simulink model "SmartphoneBatteryRectifierModel"  (R2024a)
settings: Solver=ode23t  StartTime=0.0  StopTime=10  RelTol=1e-3
libraries: nesl_utility x8, fl_lib x6, ee_lib x4, batteryecm_lib x1
settings Model: Creator=callie  LastModifiedBy=callie
settings SimscapeCC: SimscapeLogType=all  SimscapeLogLimitData=off

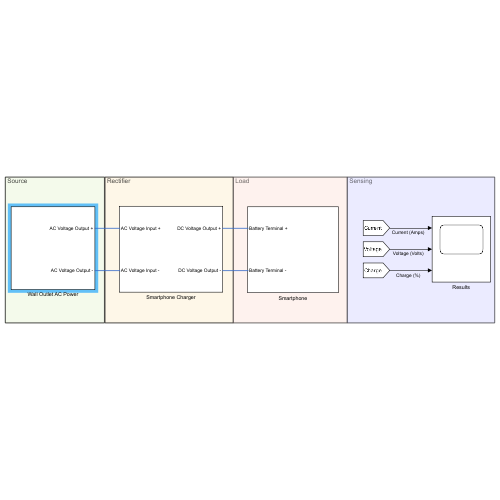
[thumbnail: Simulink's stored preview of the top-level diagram]
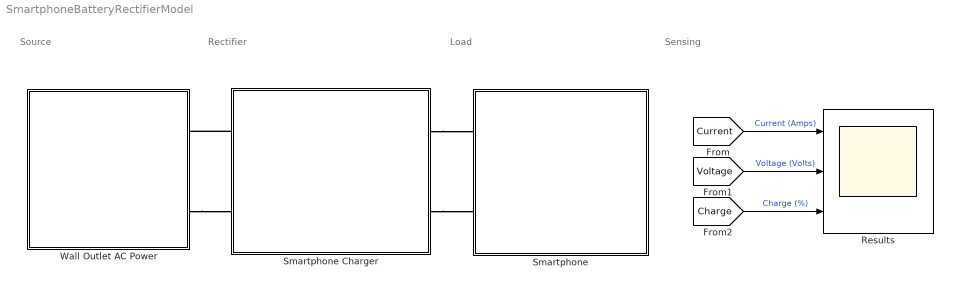
== system SmartphoneBatteryRectifierModel ==
  note: Sensing
  note: Load
  note: Rectifier
  note: Source
  Results : Scope  NumInputPorts=3
  Smartphone : Subsystem
      settings: PortSchema="{\"entries\":[{\"content\":{\"sides\":[{\"content\":{},\"type\":\"ConnectorPlacement.EquallySpacedRectSide\",\"uuid\":\"c6623932-9384-4505-9c8a-7aa7c6d03efe\"},{\"content\":{\"side\":\"RIGHT\"},\"type\":\"ConnectorPlacement.EquallySpacedRectSide\",\"uuid\":\"b63081fa-6f2e-4d52-89b7-0b15c2ff5a8a\"},{\"content\":{\"connectorIds\":[\"LConn1\",\"LConn2\"],\"side\":\"TOP\"},\"type\":\"ConnectorPlacement.EquallySpacedRectSide\",\"uuid\":\"293a2b80-333e-46a9-baf9-140dd0ae167b\"}]},\"type\":\"ConnectorPlacement.EquallySpacedConnector\",\"uuid\":\"b1957f8b-46fc-490a-ae52-971fc17beee3\"}],\"packageUris\":[\"http://schema.mathworks.com/mf0/Connector/R2020b\"],\"version\":\"1.0\"}"
  Smartphone Charger : Subsystem
  Wall Outlet AC Power : Subsystem
      settings: PortSchema="{\"entries\":[{\"content\":{\"sides\":[{\"content\":{},\"type\":\"ConnectorPlacement.EquallySpacedRectSide\",\"uuid\":\"c6623932-9384-4505-9c8a-7aa7c6d03efe\"},{\"content\":{\"side\":\"RIGHT\"},\"type\":\"ConnectorPlacement.EquallySpacedRectSide\",\"uuid\":\"b63081fa-6f2e-4d52-89b7-0b15c2ff5a8a\"},{\"content\":{\"side\":\"TOP\"},\"type\":\"ConnectorPlacement.EquallySpacedRectSide\",\"uuid\":\"293a2b80-333e-46a9-baf9-140dd0ae167b\"},{\"content\":{\"connectorIds\":[\"RConn1\",\"RConn2\"],\"side\":\"BOTTOM\"},\"type\":\"ConnectorPlacement.EquallySpacedRectSide\",\"uuid\":\"5c4d294a-cecf-4357-a6de-56f8bde29aff\"}]},\"type\":\"ConnectorPlacement.EquallySpacedConnector\",\"uuid\":\"b1957f8b-46fc-490a-ae52-971fc17beee3\"}],\"packageUris\":[\"http://schema.mathworks.com/mf0/Connector/R2020b\"],\"version\":\"1.0\"}"
  wires:
  [Current] -> Results/1  "Current (Amps)"
  [Voltage] -> Results/2  "Voltage (Volts)"
  [Charge] -> Results/3  "Charge (%)"
  connections:
  Smartphone Charger/LConn1 -- Wall Outlet AC Power/RConn1
  Wall Outlet AC Power/RConn2 -- Smartphone Charger/LConn2
  Smartphone Charger/RConn1 -- Smartphone/LConn1
  Smartphone Charger/RConn2 -- Smartphone/LConn2

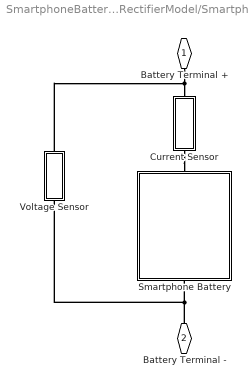
== system SmartphoneBatteryRectifierModel/Smartphone ==
  Current Sensor : Subsystem
  Smartphone Battery : Subsystem
  Voltage Sensor : Subsystem
  Battery Terminal + : PMIOPort  Side=Left
  Battery Terminal - : PMIOPort  Port=2  Side=Left
  connections:
  Battery Terminal +/RConn1 -- Voltage Sensor/LConn1 -- Current Sensor/LConn1
  Battery Terminal -/RConn1 -- Smartphone Battery/RConn1 -- Voltage Sensor/RConn1
  Current Sensor/RConn1 -- Smartphone Battery/LConn1

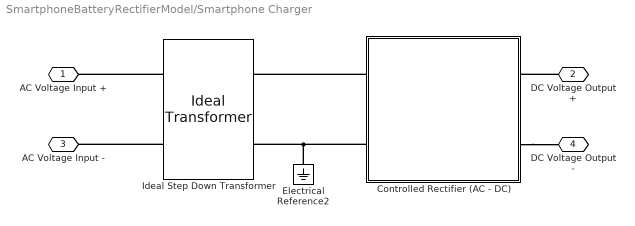
== system SmartphoneBatteryRectifierModel/Smartphone Charger ==
  Controlled Rectifier (AC - DC) : Subsystem
  Electrical Reference2 : fl_lib/Electrical/Electrical Elements/Electrical Reference
  Ideal Step Down Transformer : fl_lib/Electrical/Electrical Elements/Ideal Transformer  n=22  i1_specify=off  i1_priority=High  i1=0 A  i1_nominal_specify=off  i1_nominal_value=1  i1_nominal_unit=A  v1_specify=off  v1_priority=High  v1=0 V  v1_nominal_specify=off  v1_nominal_value=1  v1_nominal_unit=V  i2_specify=off  i2_priority=High  i2=0 A  i2_nominal_specify=off  i2_nominal_value=1  i2_nominal_unit=A  v2_specify=off  v2_priority=High  v2=0 V  v2_nominal_specify=off  v2_nominal_value=1  v2_nominal_unit=V
  AC Voltage Input + : PMIOPort  Side=Left
  DC Voltage Output + : PMIOPort  Port=2  Side=Right
  AC Voltage Input - : PMIOPort  Port=3  Side=Left
  DC Voltage Output - : PMIOPort  Port=4  Side=Right
  connections:
  Controlled Rectifier (AC - DC)/LConn1 -- Ideal Step Down Transformer/RConn1
  DC Voltage Output +/RConn1 -- Controlled Rectifier (AC - DC)/RConn1
  Controlled Rectifier (AC - DC)/LConn2 -- Electrical Reference2/LConn1 -- Ideal Step Down Transformer/RConn2
  Ideal Step Down Transformer/LConn1 -- AC Voltage Input +/RConn1
  Controlled Rectifier (AC - DC)/RConn2 -- DC Voltage Output -/RConn1
  Ideal Step Down Transformer/LConn2 -- AC Voltage Input -/RConn1

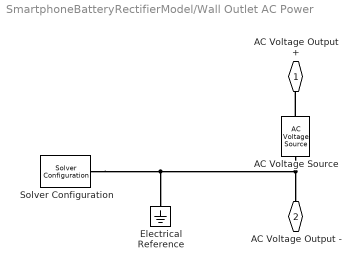
== system SmartphoneBatteryRectifierModel/Wall Outlet AC Power ==
  AC Voltage Source : fl_lib/Electrical/Electrical Sources/AC Voltage Source  amp=sqrt(2)*110 V  shift=0 deg  frequency=60 Hz
  Electrical Reference : fl_lib/Electrical/Electrical Elements/Electrical Reference
  Solver Configuration : nesl_utility/Solver Configuration  PhysicalDomain=network_engine_domain  SubClassName=solver  LeftPortType=input  RightPortType=generic  Tones=[]  Harmonics=[]  SimulateNoise=off  Profile=off  UseLocalSampling=off  EnableSwitchedLinearOptims=on  FrequencyDomain=off  UseCCode=off  RelTol=0.001  AbsTol=1e-06  MinStep=1e-09  ToWorkspace=off  RevertToSquareIcSolve=off  NumHomotopyIterations=100  PhasorMode=off  PhasorModeNumHarmonics=1  ConsistencySolver=NEWTON_FTOL  IndexReductionMethod=DerivativeReplacement  DoDC=off  ResidualTolerance=1e-09  ConsistencyTolSource=GLOBAL  ConsistencyAbsTol=0.001  ConsistencyRelTol=0.001  ConsistencyTolFactor=0.001  UseLocalSolver=off  LocalSolverChoice=NE_BACKWARD_EULER_ADVANCER  ResolveIndetEquations=on  FunctionEvalNumThread=1  LocalSolverSampleTime=0.00001  DoFixedCost=off  MaxNonlinIter=3  MaxModeIter=2  ComputeImpulses=off  ImpulseIterations=2  LinearAlgebra=auto  LinearAlgebraNumThread=0  EquationFormulation=NE_TIME_EF  DelaysMemoryBudget=1024  AutomaticFiltering=on  FilteringTimeConstant=0.001  PartitionStorageMethod=AS_NEEDED  PartitionMemoryBudget=1024  PartitionMethod=ROBUST  MultibodyUseLocalSolver=off  MultibodyLocalSolverChoice=ODE1  MultibodyLocalSolverSampleTime=0.001
  AC Voltage Output + : PMIOPort  Side=Right
  AC Voltage Output - : PMIOPort  Port=2  Side=Right
  connections:
  Solver Configuration/RConn1 -- AC Voltage Output -/RConn1 -- AC Voltage Source/RConn1 -- Electrical Reference/LConn1
  AC Voltage Source/LConn1 -- AC Voltage Output +/RConn1

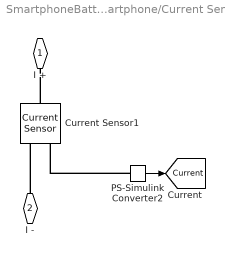
== system SmartphoneBatteryRectifierModel/Smartphone/Current Sensor ==
  Current Sensor1 : fl_lib/Electrical/Electrical Sensors/Current Sensor
  PS-Simulink Converter2 : nesl_utility/PS-Simulink Converter  PhysicalDomain=network_engine_domain  SubClassName=ps_output  LeftPortType=input  RightPortType=output  PseudoPeriodic=off  Frequencies=[]  VectorFormat=inherit  Unit=A  AffineConversion=off
  I + : PMIOPort  Side=Left
  I - : PMIOPort  Port=2  Side=Right
  tag scope: Current=global
  wires:
  PS-Simulink Converter2/1 -> [Current]
  connections:
  PS-Simulink Converter2/LConn1 -- Current Sensor1/RConn1
  Current Sensor1/LConn1 -- I +/RConn1
  I -/RConn1 -- Current Sensor1/RConn2

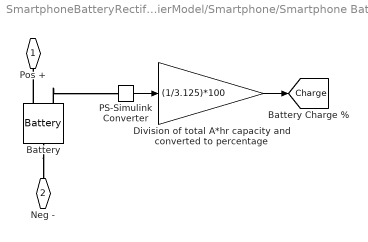
== system SmartphoneBatteryRectifierModel/Smartphone/Smartphone Battery ==
  Battery : batteryecm_lib/Battery  Vnom=4.2 V  prm_dir=simscape.enum.battery.prm_dir.disabled  R1_dis=2 Ohm  R1_ch=2 Ohm  R1=70 mOhm  prm_AH=simscape.enum.battery.prm_AH.finite  AH=3.125 A*hr  V1=3.75 V  AH1=2.753 A*hr  prm_R2=simscape.enum.battery.prm_R2.disabled  R2=2000 Ohm  Tmeas=298.15 K  charge_measurement_port=simscape.enum.battery.enable.yes  prm_dyn=simscape.enum.battery.prm_dyn.off  Rp1=0.005 Ohm  tau1=30 s  Rp2=0.005 Ohm  tau2=30 s  Rp3=0.005 Ohm  tau3=30 s  Rp4=0.005 Ohm  tau4=30 s  Rp5=0.005 Ohm  tau5=30 s  prm_fade=simscape.enum.battery.prm_fade.disabled  N_fade=100  AH_fade=45 A*hr  R1_fade=2.02 Ohm  R1_ch_fade=2.02 Ohm  V1_fade=10.35 V  prm_age=simscape.enum.battery.prm_age.disabled  prm_age_OCV=simscape.enum.battery.prm_age_OCV.OCV  OCV_age=0.9  SOC_age=60  Tmeas_age=298.15 K  delta_time_age_vec=[0] d  temperature_age_vec=[273] K  OCV_scaling_age=2.2134e6  OCV_offset_age=1.632e6  temp_exp_age=0.515833569 V  t_exp_age=0.75  Vnom_T2=12 V  R1_T2=2.2 Ohm  R1_T2_dis=2.2 Ohm  R1_T2_ch=2.2 Ohm  V1_T2=11.4 V  R2_T2=2200 Ohm  Rp1_T2=0.005 Ohm  tau1_T2=30 s  Rp2_T2=0.005 Ohm  tau2_T2=30 s  Rp3_T2=0.005 Ohm  tau3_T2=30 s  Rp4_T2=0.005 Ohm  tau4_T2=30 s  Rp5_T2=0.005 Ohm  tau5_T2=30 s  Tmeas2=273.15 K  thermal_port=simscape.enum.thermaleffects.omit  thermal_mass=30000 J/K  i_specify=off  i_priority=None  i=0 A  i_nominal_specify=off  i_nominal_value=1  i_nominal_unit=A  v_specify=off  v_priority=None  v=2.28 V  v_nominal_specify=off  v_nominal_value=22.8  v_nominal_unit=V  charge_specify=on  charge_priority=High  charge=0.78125 A*hr  charge_nominal_specify=off  charge_nominal_value=2.3  charge_nominal_unit=A*hr  num_cycles_specify=off  num_cycles_priority=High  num_cycles=0  num_cycles_nominal_specify=off  num_cycles_nominal_value=1  num_cycles_nominal_unit=1  temperature_specify=off  temperature_priority=High  temperature=298.15 K  temperature_nominal_specify=off  temperature_nominal_value=1  temperature_nominal_unit=K
      settings: LibrarySourceBlock=batt_lib/Cells/Battery  InternalSimscapePortConfiguration="{\"Bottom\":[],\"Left\":[{\"id\":\"p\",\"label\":\"+\",\"type\":\"foundation.electrical.electrical\"},{\"id\":\"q\",\"label\":\"q\",\"type\":\"output\"}],\"Right\":[{\"id\":\"n\",\"label\":\"-\",\"type\":\"foundation.electrical.electrical\"}],\"Top\":[]}"
  Division of total A*hr capacity and converted to percentage : Gain  Gain=(1/3.125)*100
  PS-Simulink Converter : nesl_utility/PS-Simulink Converter  PhysicalDomain=network_engine_domain  SubClassName=ps_output  LeftPortType=input  RightPortType=output  PseudoPeriodic=off  Frequencies=[]  VectorFormat=inherit  Unit=A*hr  AffineConversion=off
  Pos + : PMIOPort  Side=Left
  Neg - : PMIOPort  Port=2  Side=Right
  tag scope: Charge=global
  wires:
  PS-Simulink Converter/1 -> Division of total A*hr capacity and converted to percentage/1
  Division of total A*hr capacity and converted to percentage/1 -> [Charge]
  connections:
  Battery/LConn1 -- Pos +/RConn1
  Battery/RConn1 -- Neg -/RConn1
  Battery/LConn2 -- PS-Simulink Converter/LConn1

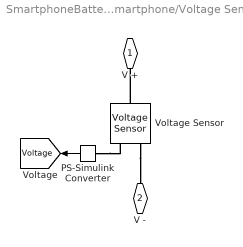
== system SmartphoneBatteryRectifierModel/Smartphone/Voltage Sensor ==
  PS-Simulink Converter : nesl_utility/PS-Simulink Converter  PhysicalDomain=network_engine_domain  SubClassName=ps_output  LeftPortType=input  RightPortType=output  PseudoPeriodic=off  Frequencies=[]  VectorFormat=inherit  Unit=V  AffineConversion=off
  Voltage Sensor : fl_lib/Electrical/Electrical Sensors/Voltage Sensor
  V + : PMIOPort  Side=Left
  V - : PMIOPort  Port=2  Side=Right
  tag scope: Voltage=global
  wires:
  PS-Simulink Converter/1 -> [Voltage]
  connections:
  PS-Simulink Converter/LConn1 -- Voltage Sensor/RConn1
  Voltage Sensor/RConn2 -- V -/RConn1
  Voltage Sensor/LConn1 -- V +/RConn1

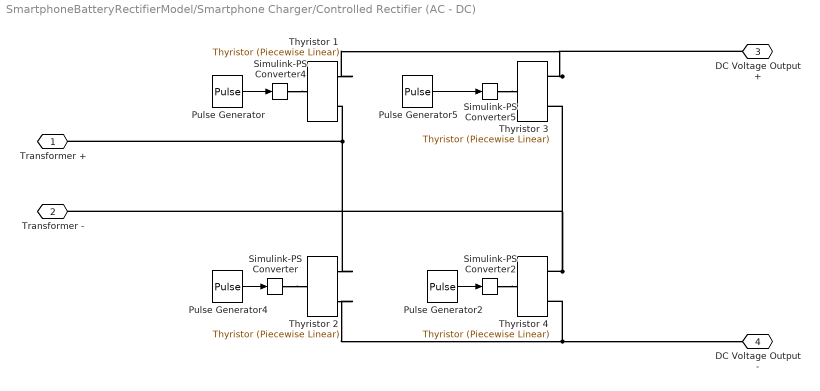
== system SmartphoneBatteryRectifierModel/Smartphone Charger/Controlled Rectifier (AC - DC) ==
  Pulse Generator : DiscretePulseGenerator  PulseType=Time based  Period=0.02  PulseWidth=5  PhaseDelay=30*0.02/360
  Pulse Generator2 : DiscretePulseGenerator  PulseType=Time based  Period=0.02  PulseWidth=5  PhaseDelay=30*0.02/360
  Pulse Generator4 : DiscretePulseGenerator  PulseType=Time based  Period=0.02  PulseWidth=5  PhaseDelay=(180+30)*0.02/360
  Pulse Generator5 : DiscretePulseGenerator  PulseType=Time based  Period=0.02  PulseWidth=5  PhaseDelay=(180+30)*0.02/360
  Simulink-PS Converter{,2,4..5} (4 alike) : nesl_utility/Simulink-PS Converter  PhysicalDomain=network_engine_domain  SubClassName=ps_input  LeftPortType=input  RightPortType=output  PseudoPeriodic=off  Frequencies=[]  NoiseDistribution=none  NoiseParameters=[]  Unit=1  AffineConversion=off  FilteringAndDerivatives=provide  SimscapeFilterOrder=1  InputFilterTimeConstant=0.001  UdotUserProvided=0
  Thyristor {1..4} (4 alike) : ee_lib/Semiconductors & Converters/Thyristor (Piecewise Linear)  port_option=ee.enum.controlport.ps  Vf=0.8 V  Ron=0.001 Ohm  Goff=1e-5 1/Ohm  Vgt=0.1 V  Ih=0.1 A  diode_param=1  diode_Vf=0.8 V  diode_Ron=0.001 Ohm  diode_Goff=1e-5 1/Ohm  diode_C=50e-9 F  diode_iRM=-235 A  diode_iF=300 A  diode_idot=-50 A/us  diode_trr_param=1  diode_trr_factor=3  diode_trr=15 us  diode_Qrr=1500 s*uA  iak_specify=off  iak_priority=None  iak=0 A  iak_nominal_specify=off  iak_nominal_value=1  iak_nominal_unit=A  vak_specify=off  vak_priority=None  vak=0 V  vak_nominal_specify=off  vak_nominal_value=1  vak_nominal_unit=V  vgk_specify=off  vgk_priority=None  vgk=0 V  vgk_nominal_specify=off  vgk_nominal_value=1  vgk_nominal_unit=V  thermal_loss_option=ee.enum.converters.thermalLossOption.constantvalues  Von_data=[0, .1, .6, .8, 1, 1.3, 1.6, 2, 2.4; 0, .1, .7, 1, 1.2, 1.5, 1.9, 2.4, 2.8] V  Tj=[298.15, 398.15] K  Iout_data=[0, .1, 1, 5, 10, 20, 40, 70, 100] A  Eon_data=[0, .0024, .024, .12, .2, .48, 1.04, 2.16, 3.24; 0, .003, .03, .15, .25, .6, 1.3, 2.7, 4.05] * 1e-3 J  Tj_loss=[298.15, 398.15] K  Iout_data_loss=[0, .1, 1, 5, 10, 20, 40, 70, 100] A  Eon_scalar=22.86e-3 J  Eoff_natural_commutation=10e-3 J  Voff=300 V  Iout_scalar=600 A  onCurrentMeasDelay=1e-4 s  diodeModelType=ee.enum.converters.diodeModelType.pwl  diodeTableType=ee.enum.diode.tableType.IfMat  diode_IfMat=[.07, .12, .19, 1.75, 4.24, 7.32, 11.2; .16, .3, .72, 2.14, 4.02, 6.35, 9.12] A  diode_VfMat=[.9, 1.15, 1.25, 1.5, 1.75, 2.17, 2.6, 2.85; .58, .68, .75, 1.1, 1.38, 1.77, 2.27, 2.7] V  diode_TjVec=[25, 125] degC  diode_VfVec=[.5, .7, .9, 1.3, 1.7, 2.1, 2.5] V  diode_IfVec=[.1, .2, .5, 1, 2, 4, 7, 10] A  diode_rec_loss_model=ee.enum.diode.reverseRecoveryModel.fixed  diode_ErecVal=0 J  diode_scaleWithIandV=true  diode_ErecMat=zeros(2, 3) J  diode_TjrecVec=[298.15, 398.15] K  diode_IfrecVec=[.1, 1, 10] A  diode_IrecVal=10 A  diode_VrecVal=10 V  diode_tFilter=1 / 1000 / 100 s  thermal_network_parameterization=ee.enum.thermalNetworkTopology.external  Rth=[.08, .5] K/W  Rth_Cauer=[.08, .1, .5] K/W  Rth_Foster=[.08, .14, .22, .16] K/W  thermal_mass_parameterization=ee.enum.thermalNetwork.timeconstant  thermal_mass=[.01, .5] J/K  thermal_mass_Cauer=[.01, .1, .5] J/K  thermal_mass_Foster=[.001, .005, .05, .5] J/K  thermal_time_constant=[.001, .2] s  thermal_time_constant_Cauer=[.001, .1, .2] s  thermal_time_constant_Foster=[7e-05, .0007, .01, .08] s  thermal_mass_initial_temperatures=[25, 25] degC  thermal_mass_initial_temperatures_Cauer=[25, 25, 25] degC  junction_thermal_mass=0.01 J/K  Tvec_initial_Foster=[25, 25, 25, 25] degC  junction_temperature_specify=off  junction_temperature_priority=None  junction_temperature=25 degC  junction_temperature_nominal_specify=off  junction_temperature_nominal_value=1  junction_temperature_nominal_unit=degC  Qj_specify=off  Qj_priority=None  Qj=0 W  Qj_nominal_specify=off  Qj_nominal_value=1  Qj_nominal_unit=W  accumulatedSwitchingLosses_specify=off  accumulatedSwitchingLosses_priority=None  accumulatedSwitchingLosses=0 J
      Thyristor 1 settings: InternalSimscapePortConfiguration="{\"Bottom\":[],\"Left\":[{\"id\":\"G\",\"label\":\"\",\"type\":\"input\"}],\"Right\":[{\"id\":\"A\",\"label\":\"\",\"type\":\"foundation.electrical.electrical\"},{\"id\":\"K\",\"label\":\"\",\"type\":\"foundation.electrical.electrical\"}],\"Top\":[]}"
      Thyristor 2 settings: InternalSimscapePortConfiguration="{\"Bottom\":[],\"Left\":[{\"id\":\"G\",\"label\":\"\",\"type\":\"input\"}],\"Right\":[{\"id\":\"A\",\"label\":\"\",\"type\":\"foundation.electrical.electrical\"},{\"id\":\"K\",\"label\":\"\",\"type\":\"foundation.electrical.electrical\"}],\"Top\":[]}"
      Thyristor 3 settings: InternalSimscapePortConfiguration="{\"Bottom\":[],\"Left\":[{\"id\":\"G\",\"label\":\"\",\"type\":\"input\"}],\"Right\":[{\"id\":\"A\",\"label\":\"\",\"type\":\"foundation.electrical.electrical\"},{\"id\":\"K\",\"label\":\"\",\"type\":\"foundation.electrical.electrical\"}],\"Top\":[]}"
      Thyristor 4 settings: LogSimulationData=on  InternalSimscapePortConfiguration="{\"Bottom\":[],\"Left\":[{\"id\":\"G\",\"label\":\"\",\"type\":\"input\"}],\"Right\":[{\"id\":\"A\",\"label\":\"\",\"type\":\"foundation.electrical.electrical\"},{\"id\":\"K\",\"label\":\"\",\"type\":\"foundation.electrical.electrical\"}],\"Top\":[]}"
  Transformer + : PMIOPort  Side=Left
  Transformer - : PMIOPort  Port=2  Side=Left
  DC Voltage Output + : PMIOPort  Port=3  Side=Right
  DC Voltage Output - : PMIOPort  Port=4  Side=Right
  wires:
  Pulse Generator5/1 -> Simulink-PS Converter5/1
  Pulse Generator4/1 -> Simulink-PS Converter/1
  Pulse Generator/1 -> Simulink-PS Converter4/1
  Pulse Generator2/1 -> Simulink-PS Converter2/1
  connections:
  Thyristor 3/RConn2 -- Thyristor 1/RConn2 -- DC Voltage Output +/RConn1
  Thyristor 2/RConn2 -- Thyristor 1/RConn1 -- Transformer +/RConn1
  Simulink-PS Converter/RConn1 -- Thyristor 2/LConn1
  Simulink-PS Converter5/RConn1 -- Thyristor 3/LConn1
  Thyristor 4/RConn2 -- Thyristor 3/RConn1 -- Transformer -/RConn1
  Simulink-PS Converter4/RConn1 -- Thyristor 1/LConn1
  Simulink-PS Converter2/RConn1 -- Thyristor 4/LConn1
  Thyristor 2/RConn1 -- Thyristor 4/RConn1 -- DC Voltage Output -/RConn1
